simulink model "M02_Baseline_Stanley"  (R2025b)
settings: Solver=ode4  StartTime=0.01  StopTime=t_sim_stop  RelTol=1e-3
undefined symbols (not defined in the file): a, b, k, L, mass, path_waypoints, v_ref_array
libraries: simulink x2, autolibshared x1
settings Model: Creator=Legion  LastModifiedBy=Legion

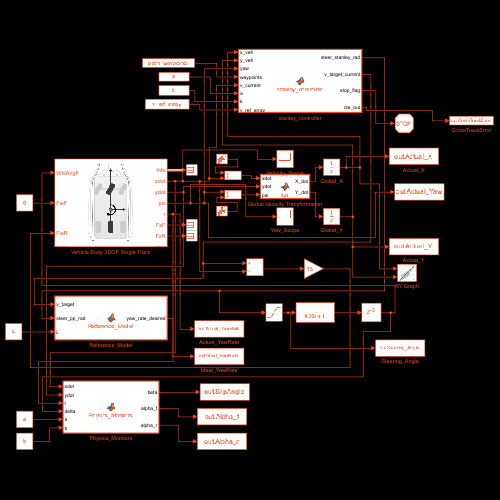
[thumbnail: Simulink's stored preview of the top-level diagram]
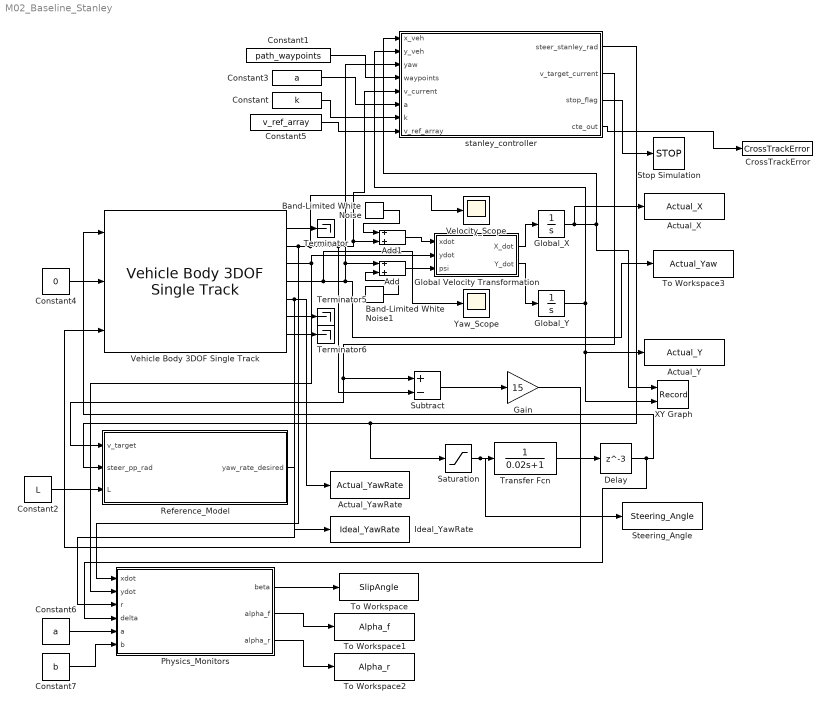
== system M02_Baseline_Stanley ==
  Actual_X : ToWorkspace  VariableName=Actual_X  SaveFormat=Timeseries  SampleTime=-1
  Actual_Y : ToWorkspace  VariableName=Actual_Y  SaveFormat=Timeseries  SampleTime=-1
  Actual_YawRate : ToWorkspace  VariableName=Actual_YawRate  SaveFormat=Timeseries  SampleTime=-1
  Add : Sum
  Add1 : Sum
  Band-Limited White Noise : simulink/Sources/Band-Limited White Noise  Cov=[0.0001]  Ts=0.01  seed=[23341]
  Band-Limited White Noise1 : simulink/Sources/Band-Limited White Noise  Cov=[0.0005]  Ts=0.01  seed=[23341]
  Constant : Constant  Value=k
  Constant1 : Constant  Value=path_waypoints
  Constant2 : Constant  Value=L
  Constant3 : Constant  Value=a
  Constant4 : Constant  Value=0
  Constant5 : Constant  Value=v_ref_array
  Constant6 : Constant  Value=a
  Constant7 : Constant  Value=b
  CrossTrackError : ToWorkspace  VariableName=CrossTrackError  SaveFormat=Timeseries  SampleTime=-1
  Delay : Delay  DelayLength=3
  Gain : Gain  Gain=15
  Global Velocity Transformation : MATLAB Function  TreatAsAtomicUnit=on
  Global_X : Integrator  InitialCondition=path_waypoints(1,1)
  Global_Y : Integrator  InitialCondition=path_waypoints(1,2)
  Ideal_YawRate : ToWorkspace  VariableName=Ideal_YawRate  SaveFormat=Timeseries  SampleTime=-1
  Physics_Monitors : MATLAB Function  TreatAsAtomicUnit=on
  Reference_Model : MATLAB Function  TreatAsAtomicUnit=on
  Saturation : Saturate  UpperLimit=30 * pi/180  LowerLimit=-30 * pi/180
  Steering_Angle : ToWorkspace  VariableName=Steering_Angle  SaveFormat=Timeseries  SampleTime=-1
  Stop Simulation : Stop
  Subtract : Sum  Inputs=+-
  Terminator : Terminator
  Terminator5 : Terminator
  Terminator6 : Terminator
  To Workspace : ToWorkspace  VariableName=SlipAngle  SaveFormat=Timeseries  SampleTime=-1
  To Workspace1 : ToWorkspace  VariableName=Alpha_f  SaveFormat=Timeseries  SampleTime=-1
  To Workspace2 : ToWorkspace  VariableName=Alpha_r  SaveFormat=Timeseries  SampleTime=-1
  To Workspace3 : ToWorkspace  VariableName=Actual_Yaw  SaveFormat=Timeseries  SampleTime=-1
  Transfer Fcn : TransferFcn  Denominator=[0.02 1]
  Vehicle Body 3DOF Single Track : autolibshared/Vehicle Body 3DOF Single Track  trackMode=Single (bicycle)  inputMode=External longitudinal forces  frontSteerMode=on  rearSteerMode=off  windMode=off  muMode=off  extFMode=off  extMMode=off  htchFMode=off  htchMMode=off  extXo=off  extpsio=off  extxdoto=off  extro=off  extYo=off  extTamb=off  extydoto=off  aMode=2  NF=2  NR=2  m=mass  a=a  b=b  h=h  dh=1  hh=0.2  X_o=0  xdot_o=0.01  CalphaMode=off  sigmaMode=off  d=0  hl=0  w=[1.4,1.4]  Cy_f=Cy_f  Cy_r=Cy_r  sigma_f=.1  sigma_r=.1  alpha_f_brk=[-0.785, -0.628, -0.471, -0.314, -0.157, 0.000, 0.157, 0.314, 0.471, 0.628, 0.785]  Cy_f_data=[2000, 3000, 4000, 5500, 7000, 9000, 7000, 5500, 4000, 3000, 2000]  alpha_r_brk=[-0.785, -0.628, -0.471, -0.314, -0.157, 0.000, 0.157, 0.314, 0.471, 0.628, 0.785]  Cy_r_data=[2000, 3000, 4000, 5500, 7000, 9000, 7000, 5500, 4000, 3000, 2000]  Y_o=0  ydot_o=0  Izz=Izz  psi_o=atan2(path_waypoints(2,2)-path_waypoints(1,2), path_waypoints(2,1)-path_waypoints(1,1))  r_o=0  Af=Af  Cd=.3  Cl=.1  Cpm=.1  beta_w=[0 0.01:0.01:0.3]  Cs=[0 0.01:0.01:0.3]  Cym=[0 1e-6:0.01:0.3]  Pabs=101325  Tair=273  g=9.81  mu=mu  xdot_tol=.01  Fznom=Fznom  Fxtire_sat=7e4  Fytire_sat=7e4  longOff=0  latOff=0  vertOff=0  wrapAng=off
  Velocity_Scope : Scope
      settings: ActiveDisplayYMinimum=0.7024131164666485  ActiveDisplayYMaximum=1.4316639746586821
  XY Graph : Record  NumPorts=2.0  FileSettingsInternal="{\"entries\":[{\"content\":{\"excelSettings\":{\"content\":{},\"type\":\"Streamout.ExcelSettings\"},\"parquetSettings\":{\"content\":{},\"type\":\"Streamout.ParquetSettings\"}},\"type\":\"Streamout.FileSettingStorage\",\"uuid\":\"\"}],\"packageUris\":[\"http:\\/\\/schema.mathworks.com\\/mf0\\/streamout_blocks\\/R2020a\"],\"version\":\"1.0\"}"  FrameSettings=[0, 0]  Layout=[1 1]  SignalsInternal="{\"entries\":[{\"content\":{\"signals\":[{\"content\":{\"blockPath\":[],\"dimensions\":[1],\"domain\":\"\",\"lineColor\":\"#4dbeee\",\"lineWidth\":2,\"port\":1,\"sid\":[\"\"],\"signalID\":1,\"signalName\":\"Global_X\"},\"type\":\"RecordBlkView.Signal\",\"uuid\":\"\"},{\"content\":{\"blockPath\":[],\"dimensions\":[1],\"domain\":\"\",\"lineColor\":\"#a2142f\",\"lineWidth\":2,\"port\":2,\"sid\":[\"\"],\"signalID\":2,\"signalName\":\"Global_Y\"},\"type\":\"RecordBlkView.Signal\",\"uuid\":\"\"}]},\"type\":\"RecordBlkView.InputSignals\",\"uuid\":\"\"}],\"packageUris\":[\"http:\\/\\/schema.mathworks.com\\/mf0\\/streamout_blocks\\/R2020a\"],\"version\":\"1.0\"}"  VisualizationBindings="{\"xyplotplugin\":{\"info\":[{\"series\":[],\"subplotID\":1}]}}"  CompatibilityTag=XY
  Yaw_Scope : Scope
      settings: ActiveDisplayYMinimum=-0.24426851447788056  ActiveDisplayYMaximum=1.1237341178679363
  stanley_controller : MATLAB Function  TreatAsAtomicUnit=on
  wires:
  Constant1/1 -> stanley_controller/4(waypoints)
  Subtract/1 -> Gain/1
  Gain/1 -> Vehicle Body 3DOF Single Track/3
  Vehicle Body 3DOF Single Track/3 -> Global Velocity Transformation/2(ydot), Physics_Monitors/2(ydot)
  stanley_controller/1(steer_stanley_rad) -> Saturation/1, Reference_Model/2(steer_pp_rad)
  Vehicle Body 3DOF Single Track/7 -> Terminator6/1
  Vehicle Body 3DOF Single Track/2 -> Physics_Monitors/1(xdot), Velocity_Scope/1, Add1/2, stanley_controller/5(v_current), Subtract/2
  Saturation/1 -> Steering_Angle/1, Transfer Fcn/1
  Constant3/1 -> stanley_controller/6(a)
  Vehicle Body 3DOF Single Track/1 -> Terminator/1
  Vehicle Body 3DOF Single Track/4 -> Yaw_Scope/1, To Workspace3/1, Add/1, stanley_controller/3(yaw)
  Global Velocity Transformation/2(Y_dot) -> Global_Y/1
  Transfer Fcn/1 -> Delay/1
  Global_Y/1 -> XY Graph/2, Actual_Y/1, stanley_controller/2(y_veh)
  Reference_Model/1(yaw_rate_desired) -> Ideal_YawRate/1
  Global Velocity Transformation/1(X_dot) -> Global_X/1
  Global_X/1 -> Actual_X/1, stanley_controller/1(x_veh), XY Graph/1
  Constant4/1 -> Vehicle Body 3DOF Single Track/2
  Vehicle Body 3DOF Single Track/6 -> Terminator5/1
  Vehicle Body 3DOF Single Track/5 -> Physics_Monitors/3(r), Actual_YawRate/1
  stanley_controller/2(v_target_current) -> Reference_Model/1(v_target), Subtract/1
  Constant5/1 -> stanley_controller/8(v_ref_array)
  Constant/1 -> stanley_controller/7(k)
  Constant2/1 -> Reference_Model/3(L)
  Constant6/1 -> Physics_Monitors/5(a)
  Constant7/1 -> Physics_Monitors/6(b)
  Physics_Monitors/1(beta) -> To Workspace/1
  Physics_Monitors/2(alpha_f) -> To Workspace1/1
  Physics_Monitors/3(alpha_r) -> To Workspace2/1
  stanley_controller/3(stop_flag) -> Stop Simulation/1
  Band-Limited White Noise/1 -> Add1/1
  Add1/1 -> Global Velocity Transformation/1(xdot)
  Band-Limited White Noise1/1 -> Add/2
  Add/1 -> Global Velocity Transformation/3(psi)
  Delay/1 -> Physics_Monitors/4(delta), Vehicle Body 3DOF Single Track/1
  stanley_controller/4(cte_out) -> CrossTrackError/1

== matlab function M02_Baseline_Stanley/stanley_controller ==
  settings: updateMethod=DISCRETE
  data: x_veh input; steer_stanley_rad output; y_veh input; yaw input; waypoints input; v_current input; a input; k input; v_target_current output; v_ref_array input; stop_flag output; cte_out output
function [steer_stanley_rad, v_target_current, stop_flag, cte_out] = stanley_controller(x_veh, y_veh, yaw, waypoints, v_current, a, k, v_ref_array)
    persistent has_finished last_closest_idx;
    if isempty(has_finished), has_finished = false; end
    if isempty(last_closest_idx), last_closest_idx = 1; end
    
    stop_flag = 0; % Default to not stopping
    
    % 1. The Finish Line Logic
    if last_closest_idx > (length(waypoints) * 0.95)
        dx_track = waypoints(end, 1) - waypoints(end-1, 1);
        dy_track = waypoints(end, 2) - waypoints(end-1, 2);
        dx_car = x_veh - waypoints(end, 1);
        dy_car = y_veh - waypoints(end, 2);
        if (dx_track * dx_car + dy_track * dy_car) > 0
            has_finished = true;
        end
    end
    
    if has_finished
        % THE FIX: cte_out MUST be assigned a value here before returning!
        steer_stanley_rad = 0; v_target_current = 0; stop_flag = 1; cte_out = 0; 
        return; 
    end
    
    % 2. Project CG to Front Axle
    x_fa = x_veh + a * cos(yaw);
    y_fa = y_veh + a * sin(yaw);
    
    % 3. Find Closest Waypoint to Front Axle
    min_dist = inf; closest_idx = last_closest_idx;
    for i = last_closest_idx:(size(waypoints, 1) - 1)
        d = sqrt((waypoints(i,1) - x_fa)^2 + (waypoints(i,2) - y_fa)^2);
        if d < min_dist
            min_dist = d; closest_idx = i;
        end
    end
    last_closest_idx = closest_idx; 
    v_target_current = v_ref_array(closest_idx);
    
    % 4. Path Heading (yaw_path)
    dx = waypoints(closest_idx+1, 1) - waypoints(closest_idx, 1);
    dy = waypoints(closest_idx+1, 2) - waypoints(closest_idx, 2);
    yaw_path = atan2(dy, dx);
    
    % 5. Heading Error (psi_e)
    psi_e = yaw_path - yaw;
    psi_e = atan2(sin(psi_e), cos(psi_e));
    
    % 6. Cross-Track Error (e_fa) via Orthogonal Projection
    path_vec_x = dx; path_vec_y = dy;
    car_vec_x = x_fa - waypoints(closest_idx, 1);
    car_vec_y = y_fa - waypoints(closest_idx, 2);
    l2 = path_vec_x^2 + path_vec_y^2;
    if l2 > 0
        t = (car_vec_x * path_vec_x + car_vec_y * path_vec_y) / l2;
        t = max(0, min(1, t));
        proj_x = waypoints(closest_idx, 1) + t * path_vec_x;
        proj_y = waypoints(closest_idx, 2) + t * path_vec_y;
    else
        proj_x = waypoints(closest_idx, 1); proj_y = waypoints(closest_idx, 2);
    end
    
    e_fa_mag = sqrt((x_fa - proj_x)^2 + (y_fa - proj_y)^2);
    cross_prod = path_vec_x * (y_fa - waypoints(closest_idx, 2)) - path_vec_y * (x_fa - waypoints(closest_idx, 1));
    e_fa = -sign(cross_prod) * e_fa_mag;
    
    % Export CTE to workspace
    cte_out = e_fa;
    
    % 7. The Stanley Control Law
    k_soft = 0.1; 
    steer_stanley_rad = psi_e + atan((k * e_fa) / (v_current + k_soft));
    
    % 8. Physical Steering Limit (+/- 30 degrees)
    steer_max = 30 * (pi/180); 
    if steer_stanley_rad > steer_max, steer_stanley_rad = steer_max;
    elseif steer_stanley_rad < -steer_max, steer_stanley_rad = -steer_max; end
end

== matlab function M02_Baseline_Stanley/Global Velocity Transformation ==
  data: xdot input; X_dot output; ydot input; psi input; Y_dot output
function [X_dot, Y_dot] = fcn(xdot, ydot, psi)
    % Rotate Body Velocities into Global Map Velocities
    % xdot = forward speed, ydot = sideways slip
    
    X_dot = xdot * cos(psi) - ydot * sin(psi);
    Y_dot = xdot * sin(psi) + ydot * cos(psi);
end

== matlab function M02_Baseline_Stanley/Reference_Model ==
  data: v_target input; yaw_rate_desired output; steer_pp_rad input; L input
function yaw_rate_desired = Reference_Model(v_target, steer_pp_rad, L)
    % Calculate the ideal yaw rate based on Pure Pursuit steering
    yaw_rate_desired = (v_target / L) * tan(steer_pp_rad);
end

== matlab function M02_Baseline_Stanley/Physics_Monitors ==
  data: xdot input; beta output; ydot input; r input; delta input; a input; b input; alpha_f output; alpha_r output
function [beta, alpha_f, alpha_r] = Physics_Monitors(xdot, ydot, r, delta, a, b)
    % This block mathematically derives the slip angles to prove tire saturation.
    % xdot: Longitudinal velocity (m/s)
    % ydot: Lateral velocity (m/s)
    % r: Yaw rate (rad/s)
    % delta: Actual front wheel steering angle (rad)
    % a, b: Distances from CG to front/rear axles (m)

    % 1. Safety limit to prevent division by zero when starting from a standstill
    v_x_safe = max(xdot, 0.1); 

    % 2. Vehicle Slip Angle (\beta)
    % Angle between the vehicle's longitudinal axis and its actual direction of travel
    beta = atan(ydot / v_x_safe);

    % 3. Front Tire Slip Angle (\alpha_f)
    % Combines lateral velocity, yaw rotation effect (a*r), and subtracts steering angle
    alpha_f = atan((ydot + a * r) / v_x_safe) - delta;

    % 4. Rear Tire Slip Angle (\alpha_r)
    % Combines lateral velocity and yaw rotation effect (rear axle moves opposite to front during yaw)
    alpha_r = atan((ydot - b * r) / v_x_safe);
end
